simulink model "simulation"  (R2020a)
settings: Solver=VariableStepAuto  StartTime=0.0  StopTime=20  RelTol=1e-3
values from neighbouring files (symbols this model uses):
  A = [0 1; -1 -2]    [script.m]
  Ad = [0 w; -w 0]    [script.m]
  Ae = [A E; zeros(1,3)]    [script.m]
  B = [1; 1]    [script.m]
  Bd = [0; 0]    [script.m]
  Be = [B; 0]    [script.m]
  C = [1 2]    [script.m]
  Cd = [1 0]    [script.m]
  Ce = [C 0]    [script.m]
  d0 = [1; 1]    [script.m]
  E = [1; -3]    [script.m]
  G = [1; 1]    [script.m]
  hat_0 = [0; 0; 0; 0]    [script.m]
  L = (place(A_OL',C',Poles))'    [script.m]
  Le = (place(Ae',Ce',PLe))'    [script.m]
  N = 0    [script.m]
  RV = 0.01    [script.m]
undefined symbols (not defined in the file or in its folder): Continuous, L_LQE, Time
libraries: simulink x2, ctrlSharedLib x1
settings Model: Creator=hp  LastModifiedBy=hp

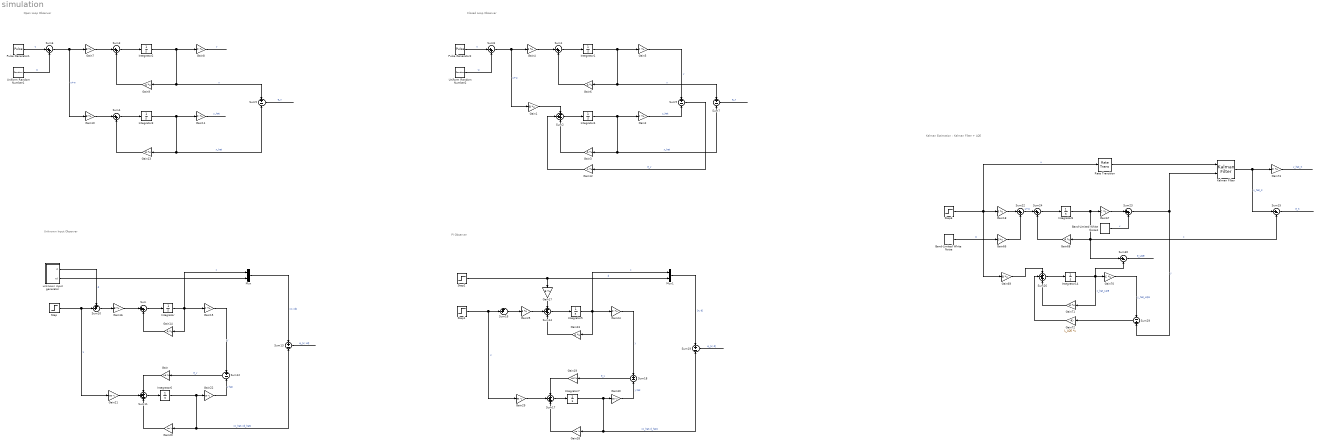
== system simulation ==
  note: Closed Loop Observer
  note: Open Loop Observer
  note: Unknown Input Observer
  note: PI Observer
  note: Kalman Estimation : Kalman Filter + LQE
  Band-Limited White Noise : simulink/Sources/Band-Limited White Noise  Cov=[0.01]  Ts=0.1  seed=[23341]
  Band-Limited White Noise1 : simulink/Sources/Band-Limited White Noise  Cov=[0.1]  Ts=0.1  seed=[23341]
  Gain : Gain  Gain=Le  Multiplication=Matrix(K*u)
  Gain{1,4,7,10,16,18,25,69} (8 alike) : Gain  Gain=B  Multiplication=Matrix(K*u)
  Gain{2,5,8,11,15,24,67,70,73} (9 alike) : Gain  Gain=C  Multiplication=Matrix(K*u)
  Gain12 : Gain  Gain=L  Multiplication=Matrix(K*u)
  Gain{3,6,9,13..14,23,68,71} (8 alike) : Gain  Gain=A  Multiplication=Matrix(K*u)
  Gain17 : Gain  Gain=E  Multiplication=Matrix(K*u)
  Gain19 : Gain  Gain=Le  Multiplication=Matrix(K*u)
  Gain20 : Gain  Gain=Ae  Multiplication=Matrix(K*u)
  Gain21 : Gain  Gain=Be  Multiplication=Matrix(K*u)
  Gain22 : Gain  Gain=Ce  Multiplication=Matrix(K*u)
  Gain28 : Gain  Gain=Ae  Multiplication=Matrix(K*u)
  Gain29 : Gain  Gain=Be  Multiplication=Matrix(K*u)
  Gain30 : Gain  Gain=Ce  Multiplication=Matrix(K*u)
  Gain66 : Gain  Gain=G  Multiplication=Matrix(K*u)
  Gain72 : Gain  Gain=L_LQE  Multiplication=Matrix(K*u)
  Integrator{,3..5,14} (5 alike) : Integrator  InitialCondition=[1; 1]
  Integrator1 : Integrator  InitialCondition=[5; 5]
  Integrator2 : Integrator  InitialCondition=[5; 5]
  Integrator6 : Integrator  InitialCondition=hat_0
  Integrator7 : Integrator  InitialCondition=[0; 0; 0]
  Integrator8 : Integrator  InitialCondition=[5; 5]
  Kalman Filter : ctrlSharedLib/Kalman Filter  TimeDomain=Continuous-Time  UseCurrentEstimator=on  ModelSource=Individual A, B, C, D matrices  ModelSourceVariable=sys  A=[0 1; -1 -2]  B=[1; 1]  C=[1 2]  D=0  NumberOfStates=2  NumberOfInputs=2  NumberOfOutputs=2  InitialEstimateSource=Dialog  X0=[1; 1]  P0=10  UseK=off  UseGH=on  NumberOfProcessNoiseInputs=2  G=G  TimeInvariantG=on  H=H  TimeInvariantH=on  Q=QW  TimeInvariantQ=on  R=RV  TimeInvariantR=on  N=N  TimeInvariantN=on  AddInputPort=on  AddEnablePort=off  OutputEstimatedY=off  OutputP=off  Ts=-1
  Mux : Mux  Inputs=2
  Mux1 : Mux  Inputs=2
  Pulse Generator1 : DiscretePulseGenerator  PulseType=Time based  Period=10  PulseWidth=50
  Pulse Generator2 : DiscretePulseGenerator  PulseType=Time based  Period=10  PulseWidth=50
  Rate Transition : RateTransition
  Step : Step  Time=0  After=0  SampleTime=0
  Step1 : Step  Time=0  After=0  SampleTime=0
  Step2 : Step  Time=0  SampleTime=0
  Step6 : Step  Time=0  SampleTime=0
  Sum{,1,3..4,6,8,22..24} (9 alike) : Sum  Inputs=|++
  Sum10 : Sum  Inputs=++|
  Sum{2,11,14,17,26} (5 alike) : Sum  Inputs=+++
  Sum{5,7,9,12..13,18..19} (7 alike) : Sum  Inputs=+-
  Sum15 : Sum  Inputs=|+-
  Sum16 : Sum  Inputs=++|
  Sum29 : Sum  Inputs=-+
  Sum30 : Sum  Inputs=|+-
  Uniform Random Number1 : UniformRandomNumber  SampleTime=0.01
  Uniform Random Number2 : UniformRandomNumber  SampleTime=0.01
  unknown input generator : Subsystem
  wires:
  Gain9/1 -> Sum3/2
  Gain10/1 -> Sum4/1
  Integrator2/1 -> Gain9/1, Sum5/1, Gain8/1  "x"
  Gain7/1 -> Sum3/1
  Gain13/1 -> Sum4/2
  Integrator3/1 -> Sum5/2, Gain13/1, Gain11/1  "x_hat"
  Uniform Random Number1/1 -> Sum6/2  "w"
  Sum6/1 -> Gain10/1, Gain7/1  "u+w"
  Sum3/1 -> Integrator2/1
  Pulse Generator1/1 -> Sum6/1  "u"
  Sum4/1 -> Integrator3/1
  Sum5/1 -> ?  "e_x"
  Gain8/1 -> ?  "y"
  Gain11/1 -> ?  "y_hat"
  Gain5/1 -> Sum9/1  "y"
  Sum2/1 -> Integrator4/1
  Pulse Generator2/1 -> Sum8/1  "u"
  Sum7/1 -> ?  "e_x"
  Gain6/1 -> Sum1/2
  Sum1/1 -> Integrator1/1
  Gain4/1 -> Sum1/1
  Integrator1/1 -> Gain6/1, Sum7/1, Gain5/1  "x"
  Sum8/1 -> Gain1/1, Gain4/1  "u+w"
  Gain1/1 -> Sum2/1
  Gain2/1 -> Sum9/2  "y_hat"
  Integrator4/1 -> Sum7/2, Gain3/1, Gain2/1  "x_hat"
  Uniform Random Number2/1 -> Sum8/2  "w"
  Sum9/1 -> Gain12/1  "e_y"
  Gain3/1 -> Sum2/3
  Gain12/1 -> Sum2/2
  unknown input generator/2(xd) -> Mux/2
  Integrator/1 -> Mux/1, Gain14/1, Gain15/1  "x"
  Step/1 -> Gain21/1, Sum10/2  "u"
  unknown input generator/1(d) -> Sum10/1  "d"
  Gain16/1 -> Sum/1
  Gain15/1 -> Sum12/1  "y"
  Gain/1 -> Sum11/1
  Sum/1 -> Integrator/1
  Mux/1 -> Sum13/1  "[x; xd]"
  Gain14/1 -> Sum/2
  Integrator6/1 -> Gain22/1, Sum13/2, Gain20/1  "[x_hat; xd_hat]"
  Gain22/1 -> Sum12/2  "y hat"
  Sum11/1 -> Integrator6/1
  Sum13/1 -> ?  "e_[x; xd]"
  Gain21/1 -> Sum11/2
  Sum10/1 -> Gain16/1
  Gain20/1 -> Sum11/3
  Sum12/1 -> Gain/1  "e_y"
  Gain17/1 -> Sum14/1
  Sum14/1 -> Integrator5/1
  Gain25/1 -> Sum14/2
  Gain24/1 -> Sum18/1  "y"
  Gain30/1 -> Sum18/2  "y hat"
  Gain29/1 -> Sum17/2
  Step2/1 -> Gain17/1, Mux1/2  "d"
  Sum18/1 -> Gain19/1  "e_y"
  Sum17/1 -> Integrator7/1
  Gain19/1 -> Sum17/1
  Mux1/1 -> Sum19/1  "[x; d]"
  Integrator5/1 -> Mux1/1, Gain23/1, Gain24/1  "x"
  Sum19/1 -> ?  "e_[x; d]"
  Gain28/1 -> Sum17/3
  Step1/1 -> Gain29/1, Sum16/2  "u"
  Sum16/1 -> Gain25/1
  Integrator7/1 -> Gain30/1, Sum19/2, Gain28/1  "[x_hat; d_hat]"
  Gain23/1 -> Sum14/3
  Gain69/1 -> Sum26/1
  Band-Limited White Noise1/1 -> Sum23/2  "v"
  Integrator8/1 -> Sum15/2, Sum30/1, Gain68/1, Gain67/1  "x"
  Gain73/1 -> ?  "y_hat_K"
  Kalman Filter/1 -> Sum15/1, Gain73/1  "x_hat_K"
  Sum26/1 -> Integrator14/1
  Sum29/1 -> Gain72/1
  Rate Transition/1 -> Kalman Filter/1
  Gain72/1 -> Sum26/2
  Gain66/1 -> Sum22/2
  Gain67/1 -> Sum23/1
  Sum24/1 -> Integrator8/1
  Sum22/1 -> Sum24/1  "u+w"
  Step6/1 -> Gain69/1, Rate Transition/1, Gain18/1  "u"
  Gain18/1 -> Sum22/1
  Band-Limited White Noise/1 -> Gain66/1  "w"
  Gain68/1 -> Sum24/2
  Gain71/1 -> Sum26/3
  Sum30/1 -> ?  "e_LQE"
  Integrator14/1 -> Gain70/1, Sum30/2, Gain71/1  "x_hat_LQE"
  Sum15/1 -> ?  "e_K"
  Gain70/1 -> Sum29/1  "y_hat_LQE"
  Sum23/1 -> Sum29/2, Kalman Filter/2  "y"

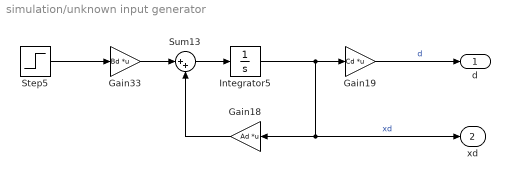
== system simulation/unknown input generator ==
  Gain18 : Gain  Gain=Ad  Multiplication=Matrix(K*u)
  Gain19 : Gain  Gain=Cd  Multiplication=Matrix(K*u)
  Gain33 : Gain  Gain=Bd  Multiplication=Matrix(K*u)
  Integrator5 : Integrator  InitialCondition=d0
  Step5 : Step  Time=0  After=0  SampleTime=0
  Sum13 : Sum  Inputs=|++
  d : Outport
  xd : Outport  Port=2
  wires:
  Integrator5/1 -> Gain18/1, xd/1, Gain19/1  "xd"
  Gain19/1 -> d/1  "d"
  Step5/1 -> Gain33/1
  Gain18/1 -> Sum13/2
  Gain33/1 -> Sum13/1
  Sum13/1 -> Integrator5/1
